simulink model "lala"  (R2017a)
settings: Solver=VariableStepAuto  StartTime=0.0  StopTime=10.0  RelTol=1e-3
settings Model: Creator=Felipe  LastModifiedBy=Felipe

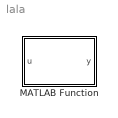
== system lala ==
  MATLAB Function : MATLAB Function  TreatAsAtomicUnit=on

== matlab function lala/MATLAB Function ==
  data: u input; y output
function y = fcn(u)
coder.extrinsic('opcua');
coder.extrinsic('connect');
ua_client = opcua('opc.tcp://localhost:4840/freeopcua/server/');
connect(ua_client);
y = u;
